simulink model "SimpleControl"  (R2019a)
settings: Solver=VariableStepAuto  StartTime=0.0  StopTime=12  RelTol=1e-3
values from neighbouring files (symbols this model uses):
  Ar = 0.250*0.106    (= 0.0265)    [init.m]
  b = 72e-6    (= 7.2e-05)    [init.m]
  Cd = 1    [init.m]
  d = 1.1e-5    (= 1.1e-05)    [init.m]
  g = 9.80665    [init.m]
  Ix = 1e-3    (= 0.001)    [init.m]
  Iy = 1e-3    (= 0.001)    [init.m]
  Iz = 2e-3    (= 0.002)    [init.m]
  Jm = 3.4e-5    (= 3.4e-05)    [init.m]
  l = 0.12    [init.m]
  m = 0.46    [init.m]
  p = 1.225    [init.m]
  T2AV = 31.5    [init.m]
undefined symbols (not defined in the file or in its folder): magnitude
libraries: simulink x4
settings Model: Creator=Amador  LastModifiedBy=Amador

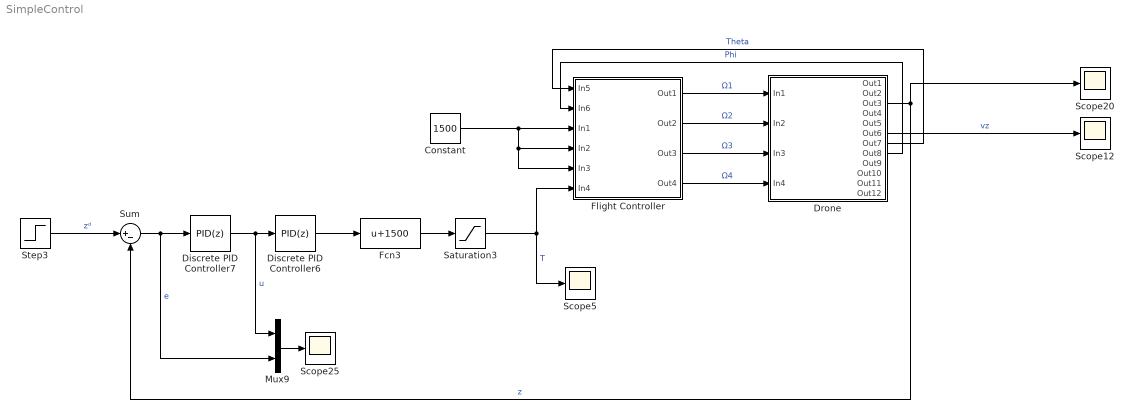
== system SimpleControl ==
  Constant : Constant  Value=1500
  Discrete PID Controller6 : simulink/Continuous/PID Controller  Controller=PID  Form=Parallel  TimeDomain=Discrete-time  SampleTime=1/60  IntegratorMethod=Forward Euler  FilterMethod=Forward Euler  ControllerParametersSource=internal  P=50  I=0.5  D=50  UseFilter=on  N=10  TunerSelectOption=Transfer Function Based (PID Tuner App)  InitialConditionSource=internal  InitialConditionForIntegrator=0  InitialConditionForFilter=0  DifferentiatorICPrevScaledInput=0  ExternalReset=none  TrackingMode=off  Kt=1  LimitOutput=off  UpperSaturationLimit=inf  LowerSaturationLimit=-inf  LinearizeAsGain=off  AntiWindupMode=none  Kb=1  POutMin=[]  POutMax=[]  IOutMin=[]  IOutMax=[]  DOutMin=[]  DOutMax=[]  NOutMin=[]  NOutMax=[]  SumOutMin=[]  SumOutMax=[]  SaturationOutMin=[]  SaturationOutMax=[]  PParamMin=[]  PParamMax=[]  IParamMin=[]  IParamMax=[]  DParamMin=[]  DParamMax=[]  NParamMin=[]  NParamMax=[]  KbParamMin=[]  KbParamMax=[]  KtParamMin=[]  KtParamMax=[]  KbOutMin=[]  KbOutMax=[]  KtOutMin=[]  KtOutMax=[]  IntegratorOutMin=[]  IntegratorOutMax=[]  FilterOutMin=[]  FilterOutMax=[]  SumI1OutMin=[]  SumI1OutMax=[]  SumI2OutMin=[]  SumI2OutMax=[]  SumI3OutMin=[]  SumI3OutMax=[]  SumI4OutMin=[]  SumI4OutMax=[]  SumDOutMin=[]  SumDOutMax=[]  DifferentiatorOutMin=[]  DifferentiatorOutMax=[]  FilterDiffOutCoefMin=[]  FilterDiffOutCoefMax=[]  ReciprocalOutMin=[]  ReciprocalOutMax=[]  SumDenOutMin=[]  SumDenOutMax=[]  SumNumOutMin=[]  SumNumOutMax=[]  DivideOutMin=[]  DivideOutMax=[]  IntegratorContinuousStateAttributes=''  IntegratorStateMustResolveToSignalObject=off  IntegratorRTWStateStorageClass=Auto  FilterContinuousStateAttributes=''  FilterStateMustResolveToSignalObject=off  FilterRTWStateStorageClass=Auto  ParallelPVariant=InternalParameters  IdealPVariant=Disabled  IVariant=InternalParameters  DVariant=InternalParameters  IntegratorVariant=Discrete  SatVariant=Disabled  AWVariant=Passthrough  PCopyVariant=Disabled  TRVariant=Disabled  FdbkBlocksVariant=Forward  IdealPFdbkVariant=Disabled  SatFdbkVariant=Disabled  DerivativeFilterVariant=ForwardEulerFilter  NVariant=InternalParameters  NCopyVariant=Disabled  FilterICVariant=InternalICsFilter  IntegratorICVariant=InternalICs  ExternalResetVariant=Disabled  TRSumVariant=Passthrough  SumFdbkVariant=Disabled  SumVariant=Sum_PID
  Discrete PID Controller7 : simulink/Continuous/PID Controller  Controller=PID  Form=Parallel  TimeDomain=Discrete-time  SampleTime=1/60  IntegratorMethod=Forward Euler  FilterMethod=Forward Euler  ControllerParametersSource=internal  P=5  I=3  D=0.5  UseFilter=on  N=10  TunerSelectOption=Transfer Function Based (PID Tuner App)  InitialConditionSource=internal  InitialConditionForIntegrator=0  InitialConditionForFilter=0  DifferentiatorICPrevScaledInput=0  ExternalReset=none  TrackingMode=off  Kt=1  LimitOutput=off  UpperSaturationLimit=inf  LowerSaturationLimit=-inf  LinearizeAsGain=off  AntiWindupMode=none  Kb=1  POutMin=[]  POutMax=[]  IOutMin=[]  IOutMax=[]  DOutMin=[]  DOutMax=[]  NOutMin=[]  NOutMax=[]  SumOutMin=[]  SumOutMax=[]  SaturationOutMin=[]  SaturationOutMax=[]  PParamMin=[]  PParamMax=[]  IParamMin=[]  IParamMax=[]  DParamMin=[]  DParamMax=[]  NParamMin=[]  NParamMax=[]  KbParamMin=[]  KbParamMax=[]  KtParamMin=[]  KtParamMax=[]  KbOutMin=[]  KbOutMax=[]  KtOutMin=[]  KtOutMax=[]  IntegratorOutMin=[]  IntegratorOutMax=[]  FilterOutMin=[]  FilterOutMax=[]  SumI1OutMin=[]  SumI1OutMax=[]  SumI2OutMin=[]  SumI2OutMax=[]  SumI3OutMin=[]  SumI3OutMax=[]  SumI4OutMin=[]  SumI4OutMax=[]  SumDOutMin=[]  SumDOutMax=[]  DifferentiatorOutMin=[]  DifferentiatorOutMax=[]  FilterDiffOutCoefMin=[]  FilterDiffOutCoefMax=[]  ReciprocalOutMin=[]  ReciprocalOutMax=[]  SumDenOutMin=[]  SumDenOutMax=[]  SumNumOutMin=[]  SumNumOutMax=[]  DivideOutMin=[]  DivideOutMax=[]  IntegratorContinuousStateAttributes=''  IntegratorStateMustResolveToSignalObject=off  IntegratorRTWStateStorageClass=Auto  FilterContinuousStateAttributes=''  FilterStateMustResolveToSignalObject=off  FilterRTWStateStorageClass=Auto  ParallelPVariant=InternalParameters  IdealPVariant=Disabled  IVariant=InternalParameters  DVariant=InternalParameters  IntegratorVariant=Discrete  SatVariant=Disabled  AWVariant=Passthrough  PCopyVariant=Disabled  TRVariant=Disabled  FdbkBlocksVariant=Forward  IdealPFdbkVariant=Disabled  SatFdbkVariant=Disabled  DerivativeFilterVariant=ForwardEulerFilter  NVariant=InternalParameters  NCopyVariant=Disabled  FilterICVariant=InternalICsFilter  IntegratorICVariant=InternalICs  ExternalResetVariant=Disabled  TRSumVariant=Passthrough  SumFdbkVariant=Disabled  SumVariant=Sum_PID
  Drone : Subsystem
  Fcn3 : Fcn  Expr=u+1500
  Flight Controller : Subsystem
  Mux9 : Mux  Inputs=2
  Saturation3 : Saturate  UpperLimit=1800  LowerLimit=1250
  Scope{5,12,20,25} (4 alike) : Scope
  Step3 : Step  Time=5  Before=5  After=5  SampleTime=0
  Sum : Sum  Inputs=|+-
  wires:
  Sum/1 -> Mux9/2, Discrete PID Controller7/1  "e"
  Drone/3(Out3) -> Sum/2, Scope20/1  "z"
  Step3/1 -> Sum/1  "zᵈ"
  Flight Controller/1(Out1) -> Drone/1(In1)  "Ω1"
  Drone/7(Out7) -> Flight Controller/1(In5)  "Theta"
  Drone/6(Out6) -> Scope12/1  "vz"
  Drone/8(Out8) -> Flight Controller/2(In6)  "Phi"
  Flight Controller/2(Out2) -> Drone/2(In2)  "Ω2"
  Flight Controller/3(Out3) -> Drone/3(In3)  "Ω3"
  Flight Controller/4(Out4) -> Drone/4(In4)  "Ω4"
  Fcn3/1 -> Saturation3/1
  Saturation3/1 -> Scope5/1, Flight Controller/6(In4)  "T"
  Discrete PID Controller6/1 -> Fcn3/1
  Discrete PID Controller7/1 -> Mux9/1, Discrete PID Controller6/1  "u"
  Mux9/1 -> Scope25/1
  Constant/1 -> Flight Controller/3(In1), Flight Controller/4(In2), Flight Controller/5(In3)

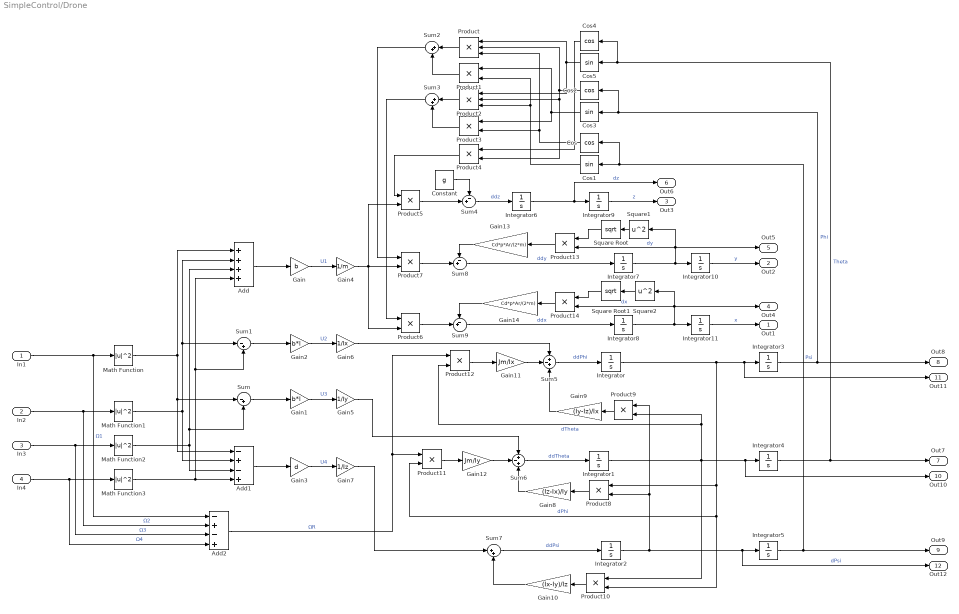
== system SimpleControl/Drone ==
  In1 : Inport
  In2 : Inport  Port=2
  In3 : Inport  Port=3
  In4 : Inport  Port=4
  Add : Sum  Inputs=++++
  Add1 : Sum  Inputs=-+-+
  Add2 : Sum  Inputs=-+-+
  Constant : Constant  Value=g
  Cos : Trigonometry  Operator=cos
  Cos1 : Trigonometry
  Cos2 : Trigonometry  Operator=cos
  Cos3 : Trigonometry
  Cos4 : Trigonometry  Operator=cos
  Cos5 : Trigonometry
  Gain : Gain  Gain=b
  Gain1 : Gain  Gain=b*l
  Gain10 : Gain  Gain=(Ix-Iy)/Iz
  Gain11 : Gain  Gain=Jm/Ix
  Gain12 : Gain  Gain=Jm/Iy
  Gain13 : Gain  Gain=Cd*p*Ar/(2*m)
  Gain14 : Gain  Gain=Cd*p*Ar/(2*m)
  Gain2 : Gain  Gain=b*l
  Gain3 : Gain  Gain=d
  Gain4 : Gain  Gain=1/m
  Gain5 : Gain  Gain=1/Iy
  Gain6 : Gain  Gain=1/Ix
  Gain7 : Gain  Gain=1/Iz
  Gain8 : Gain  Gain=(Iz-Ix)/Iy
  Gain9 : Gain  Gain=(Iy-Iz)/Ix
  Integrator{,1..11} (12 alike) : Integrator
  Math Function{,1..3} (4 alike) : Math  Operator=magnitude^2  SaturateOnIntegerOverflow=on
  Product : Product  Inputs=3
  Product{1,3..14} (13 alike) : Product
  Product2 : Product  Inputs=3
  Square Root : Sqrt  SaturateOnIntegerOverflow=on
  Square Root1 : Sqrt  SaturateOnIntegerOverflow=on
  Square1 : Math  Operator=square  SaturateOnIntegerOverflow=on
  Square2 : Math  Operator=square  SaturateOnIntegerOverflow=on
  Sum : Sum  Inputs=|-+
  Sum1 : Sum  Inputs=|-+
  Sum2 : Sum  Inputs=|++
  Sum3 : Sum  Inputs=|++
  Sum4 : Sum  Inputs=-+|
  Sum5 : Sum  Inputs=+-+
  Sum6 : Sum  Inputs=+-+
  Sum7 : Sum  Inputs=|++
  Sum8 : Sum  Inputs=-+|
  Sum9 : Sum  Inputs=-+|
  Out1 : Outport
  Out2 : Outport  Port=2
  Out3 : Outport  Port=3
  Out4 : Outport  Port=4
  Out5 : Outport  Port=5
  Out6 : Outport  Port=6
  Out7 : Outport  Port=7
  Out8 : Outport  Port=8
  Out9 : Outport  Port=9
  Out10 : Outport  Port=10
  Out11 : Outport  Port=11
  Out12 : Outport  Port=12
  wires:
  Add/1 -> Gain/1
  In1/1 -> Add2/1, Math Function/1  "Ω1"
  In2/1 -> Add2/2, Math Function1/1  "Ω2"
  In3/1 -> Add2/3, Math Function2/1  "Ω3"
  In4/1 -> Add2/4, Math Function3/1  "Ω4"
  Sum/1 -> Gain1/1
  Sum1/1 -> Gain2/1
  Add1/1 -> Gain3/1
  Gain1/1 -> Gain5/1  "U3"
  Gain2/1 -> Gain6/1  "U2"
  Gain3/1 -> Gain7/1  "U4"
  Cos5/1 -> Product2/1, Product/1
  Cos2/1 -> Product/2, Product2/2, Product4/2
  Cos/1 -> Product/3, Product3/2
  Cos3/1 -> Product3/1, Product1/1
  Cos1/1 -> Product2/3, Product1/2
  Cos4/1 -> Product4/1
  Product2/1 -> Sum3/1
  Product/1 -> Sum2/1
  Product1/1 -> Sum2/2
  Product3/1 -> Sum3/2
  Product4/1 -> Product5/1
  Sum3/1 -> Product6/1
  Sum2/1 -> Product7/1
  Gain/1 -> Gain4/1  "U1"
  Gain4/1 -> Product5/2, Product7/2, Product6/2
  Sum9/1 -> Integrator8/1  "ddx"
  Sum8/1 -> Integrator7/1  "ddy"
  Product5/1 -> Sum4/2
  Constant/1 -> Sum4/1
  Sum4/1 -> Integrator6/1  "ddz"
  Gain7/1 -> Sum7/1
  Sum5/1 -> Integrator/1  "ddPhi"
  Sum6/1 -> Integrator1/1  "ddTheta"
  Sum7/1 -> Integrator2/1  "ddPsi"
  Integrator/1 -> Out11/1, Integrator3/1, Product11/2, Product10/2, Product8/1  "dPhi"
  Integrator1/1 -> Product12/2, Product9/2, Out10/1, Integrator4/1, Product10/1  "dTheta"
  Integrator2/1 -> Out12/1, Integrator5/1, Product8/2, Product9/1  "dPsi"
  Product8/1 -> Gain8/1
  Gain8/1 -> Sum6/3
  Product9/1 -> Gain9/1
  Gain9/1 -> Sum5/3
  Product10/1 -> Gain10/1
  Gain10/1 -> Sum7/2
  Add2/1 -> Product12/1, Product11/1  "ΩR"
  Gain11/1 -> Sum5/2
  Product12/1 -> Gain11/1
  Gain12/1 -> Sum6/2
  Product11/1 -> Gain12/1
  Integrator5/1 -> Out9/1, Cos/1, Cos1/1  "Psi"
  Integrator4/1 -> Cos4/1, Cos5/1, Out7/1  "Theta"
  Integrator3/1 -> Cos2/1, Cos3/1, Out8/1  "Phi"
  Integrator8/1 -> Product14/2, Square2/1, Out4/1, Integrator11/1  "dx"
  Integrator7/1 -> Product13/2, Square1/1, Out5/1, Integrator10/1  "dy"
  Integrator6/1 -> Out6/1, Integrator9/1  "dz"
  Integrator9/1 -> Out3/1  "z"
  Integrator10/1 -> Out2/1  "y"
  Integrator11/1 -> Out1/1  "x"
  Gain6/1 -> Sum5/1
  Gain5/1 -> Sum6/1
  Math Function3/1 -> Add1/4, Add/4, Sum1/2
  Math Function2/1 -> Add/3, Sum/2, Add1/3
  Math Function1/1 -> Add/2, Sum1/1, Add1/2
  Math Function/1 -> Add/1, Add1/1, Sum/1
  Product7/1 -> Sum8/2
  Square1/1 -> Square Root/1
  Square Root/1 -> Product13/1
  Product13/1 -> Gain13/1
  Gain13/1 -> Sum8/1
  Square2/1 -> Square Root1/1
  Square Root1/1 -> Product14/1
  Product14/1 -> Gain14/1
  Product6/1 -> Sum9/2
  Gain14/1 -> Sum9/1

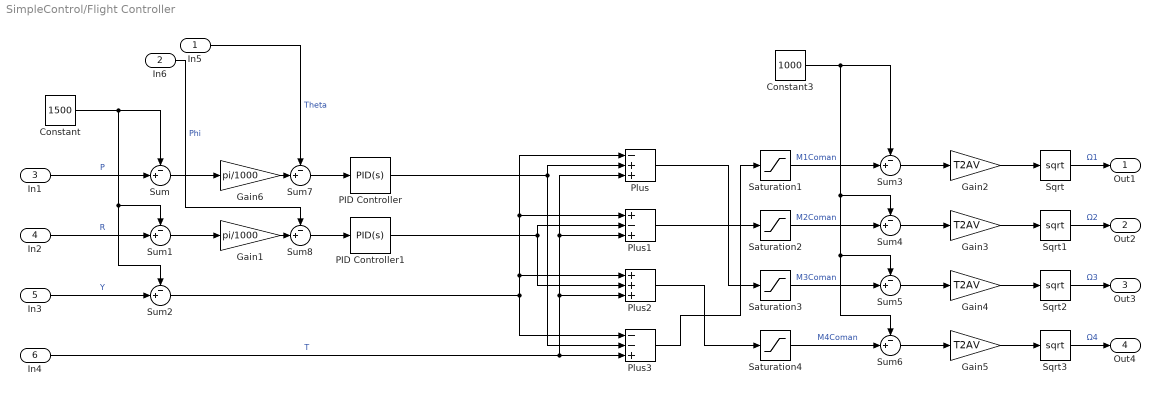
== system SimpleControl/Flight Controller ==
  In5 : Inport
  In6 : Inport  Port=2
  In1 : Inport  Port=3
  In2 : Inport  Port=4
  In3 : Inport  Port=5
  In4 : Inport  Port=6
  Constant : Constant  Value=1500
  Constant3 : Constant  Value=1000
  Gain1 : Gain  Gain=pi/1000
  Gain{2..5} (4 alike) : Gain  Gain=T2AV
  Gain6 : Gain  Gain=pi/1000
  PID Controller : simulink/Continuous/PID Controller  Controller=PID  Form=Parallel  TimeDomain=Continuous-time  SampleTime=-1  IntegratorMethod=Forward Euler  FilterMethod=Forward Euler  ControllerParametersSource=internal  P=4  I=8/128  D=6  UseFilter=on  N=100  TunerSelectOption=Transfer Function Based (PID Tuner App)  InitialConditionSource=internal  InitialConditionForIntegrator=0  InitialConditionForFilter=0  DifferentiatorICPrevScaledInput=0  ExternalReset=none  TrackingMode=off  Kt=1  LimitOutput=on  UpperSaturationLimit=50  LowerSaturationLimit=-50  LinearizeAsGain=off  AntiWindupMode=none  Kb=1  POutMin=[]  POutMax=[]  IOutMin=[]  IOutMax=[]  DOutMin=[]  DOutMax=[]  NOutMin=[]  NOutMax=[]  SumOutMin=[]  SumOutMax=[]  SaturationOutMin=[]  SaturationOutMax=[]  PParamMin=[]  PParamMax=[]  IParamMin=[]  IParamMax=[]  DParamMin=[]  DParamMax=[]  NParamMin=[]  NParamMax=[]  KbParamMin=[]  KbParamMax=[]  KtParamMin=[]  KtParamMax=[]  KbOutMin=[]  KbOutMax=[]  KtOutMin=[]  KtOutMax=[]  IntegratorOutMin=[]  IntegratorOutMax=[]  FilterOutMin=[]  FilterOutMax=[]  SumI1OutMin=[]  SumI1OutMax=[]  SumI2OutMin=[]  SumI2OutMax=[]  SumI3OutMin=[]  SumI3OutMax=[]  SumI4OutMin=[]  SumI4OutMax=[]  SumDOutMin=[]  SumDOutMax=[]  DifferentiatorOutMin=[]  DifferentiatorOutMax=[]  FilterDiffOutCoefMin=[]  FilterDiffOutCoefMax=[]  ReciprocalOutMin=[]  ReciprocalOutMax=[]  SumDenOutMin=[]  SumDenOutMax=[]  SumNumOutMin=[]  SumNumOutMax=[]  DivideOutMin=[]  DivideOutMax=[]  IntegratorContinuousStateAttributes=''  IntegratorStateMustResolveToSignalObject=off  IntegratorRTWStateStorageClass=Auto  FilterContinuousStateAttributes=''  FilterStateMustResolveToSignalObject=off  FilterRTWStateStorageClass=Auto  ParallelPVariant=InternalParameters  IdealPVariant=Disabled  IVariant=InternalParameters  DVariant=InternalParameters  IntegratorVariant=Continuous  SatVariant=Enabled  AWVariant=Passthrough  PCopyVariant=Disabled  TRVariant=Disabled  FdbkBlocksVariant=Forward  IdealPFdbkVariant=Disabled  SatFdbkVariant=Disabled  DerivativeFilterVariant=ContFilter  NVariant=InternalParameters  NCopyVariant=Disabled  FilterICVariant=InternalICsFilter  IntegratorICVariant=InternalICs  ExternalResetVariant=Disabled  TRSumVariant=Passthrough  SumFdbkVariant=Disabled  SumVariant=Sum_PID
  PID Controller1 : simulink/Continuous/PID Controller  Controller=PID  Form=Parallel  TimeDomain=Continuous-time  SampleTime=-1  IntegratorMethod=Forward Euler  FilterMethod=Forward Euler  ControllerParametersSource=internal  P=4  I=8/128  D=6  UseFilter=on  N=100  TunerSelectOption=Transfer Function Based (PID Tuner App)  InitialConditionSource=internal  InitialConditionForIntegrator=0  InitialConditionForFilter=0  DifferentiatorICPrevScaledInput=0  ExternalReset=none  TrackingMode=off  Kt=1  LimitOutput=on  UpperSaturationLimit=50  LowerSaturationLimit=-50  LinearizeAsGain=off  AntiWindupMode=none  Kb=1  POutMin=[]  POutMax=[]  IOutMin=[]  IOutMax=[]  DOutMin=[]  DOutMax=[]  NOutMin=[]  NOutMax=[]  SumOutMin=[]  SumOutMax=[]  SaturationOutMin=[]  SaturationOutMax=[]  PParamMin=[]  PParamMax=[]  IParamMin=[]  IParamMax=[]  DParamMin=[]  DParamMax=[]  NParamMin=[]  NParamMax=[]  KbParamMin=[]  KbParamMax=[]  KtParamMin=[]  KtParamMax=[]  KbOutMin=[]  KbOutMax=[]  KtOutMin=[]  KtOutMax=[]  IntegratorOutMin=[]  IntegratorOutMax=[]  FilterOutMin=[]  FilterOutMax=[]  SumI1OutMin=[]  SumI1OutMax=[]  SumI2OutMin=[]  SumI2OutMax=[]  SumI3OutMin=[]  SumI3OutMax=[]  SumI4OutMin=[]  SumI4OutMax=[]  SumDOutMin=[]  SumDOutMax=[]  DifferentiatorOutMin=[]  DifferentiatorOutMax=[]  FilterDiffOutCoefMin=[]  FilterDiffOutCoefMax=[]  ReciprocalOutMin=[]  ReciprocalOutMax=[]  SumDenOutMin=[]  SumDenOutMax=[]  SumNumOutMin=[]  SumNumOutMax=[]  DivideOutMin=[]  DivideOutMax=[]  IntegratorContinuousStateAttributes=''  IntegratorStateMustResolveToSignalObject=off  IntegratorRTWStateStorageClass=Auto  FilterContinuousStateAttributes=''  FilterStateMustResolveToSignalObject=off  FilterRTWStateStorageClass=Auto  ParallelPVariant=InternalParameters  IdealPVariant=Disabled  IVariant=InternalParameters  DVariant=InternalParameters  IntegratorVariant=Continuous  SatVariant=Enabled  AWVariant=Passthrough  PCopyVariant=Disabled  TRVariant=Disabled  FdbkBlocksVariant=Forward  IdealPFdbkVariant=Disabled  SatFdbkVariant=Disabled  DerivativeFilterVariant=ContFilter  NVariant=InternalParameters  NCopyVariant=Disabled  FilterICVariant=InternalICsFilter  IntegratorICVariant=InternalICs  ExternalResetVariant=Disabled  TRSumVariant=Passthrough  SumFdbkVariant=Disabled  SumVariant=Sum_PID
  Plus : Sum  Inputs=-++
  Plus1 : Sum  Inputs=+-+
  Plus2 : Sum  Inputs=+++
  Plus3 : Sum  Inputs=--+
  Saturation{1..4} (4 alike) : Saturate  UpperLimit=2000  LowerLimit=1000
  Sqrt{,1..3} (4 alike) : Sqrt  SaturateOnIntegerOverflow=on
  Sum{,1..8} (9 alike) : Sum  Inputs=-+|
  Out1 : Outport
  Out2 : Outport  Port=2
  Out3 : Outport  Port=3
  Out4 : Outport  Port=4
  wires:
  In1/1 -> Sum/2  "P"
  In2/1 -> Sum1/2  "R"
  In3/1 -> Sum2/2  "Y"
  In4/1 -> Plus/3, Plus1/3, Plus2/3, Plus3/3  "T"
  Constant/1 -> Sum2/1, Sum1/1, Sum/1
  PID Controller/1 -> Plus3/2, Plus/2
  PID Controller1/1 -> Plus1/2, Plus2/2
  Saturation1/1 -> Sum3/2  "M1Coman"
  Constant3/1 -> Sum6/1, Sum5/1, Sum4/1, Sum3/1
  Sum3/1 -> Gain2/1
  Saturation2/1 -> Sum4/2  "M2Coman"
  Sum4/1 -> Gain3/1
  Saturation3/1 -> Sum5/2  "M3Coman"
  Sum5/1 -> Gain4/1
  Saturation4/1 -> Sum6/2  "M4Coman"
  Sum6/1 -> Gain5/1
  Sqrt/1 -> Out1/1  "Ω1"
  Gain5/1 -> Sqrt3/1
  Gain3/1 -> Sqrt1/1
  Gain4/1 -> Sqrt2/1
  Plus3/1 -> Saturation1/1
  Plus/1 -> Saturation3/1
  Plus1/1 -> Saturation2/1
  Plus2/1 -> Saturation4/1
  Sum1/1 -> Gain1/1
  Sum/1 -> Gain6/1
  In5/1 -> Sum7/1  "Theta"
  In6/1 -> Sum8/1  "Phi"
  Sum8/1 -> PID Controller1/1
  Sum7/1 -> PID Controller/1
  Gain2/1 -> Sqrt/1
  Sqrt1/1 -> Out2/1  "Ω2"
  Sqrt2/1 -> Out3/1  "Ω3"
  Sqrt3/1 -> Out4/1  "Ω4"
  Gain6/1 -> Sum7/2
  Gain1/1 -> Sum8/2
  Sum2/1 -> Plus/1, Plus1/1, Plus2/1, Plus3/1
